simulink model "FT_CAN_messages"  (R2021b)
settings: Solver=FixedStepDiscrete  StartTime=0.0  StopTime=Inf  FixedStep=5e-2  RelTol=1e-3
model workspace (MAT data in the model file):
  MAX_UINT4 = Simulink.Parameter
  MAX_UINT4.Value = 15
  MAX_UINT4.DataType = 'auto'
  MAX_UINT4.Complexity = 'real'
  MAX_UINT4.Dimensions = [1 1]
undefined symbols (not defined in the file): canChannel
libraries: canmsglib x15, canlib x4, slrealtimesharedmemorylib x1, simulink_extras x1
settings Model: Creator=mfussi  LastModifiedBy=ngenesio

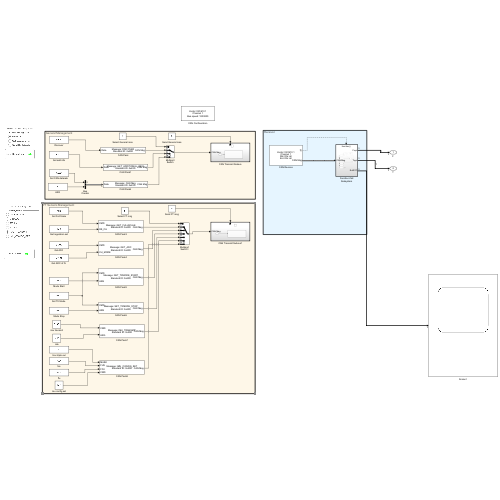
[thumbnail: Simulink's stored preview of the top-level diagram]
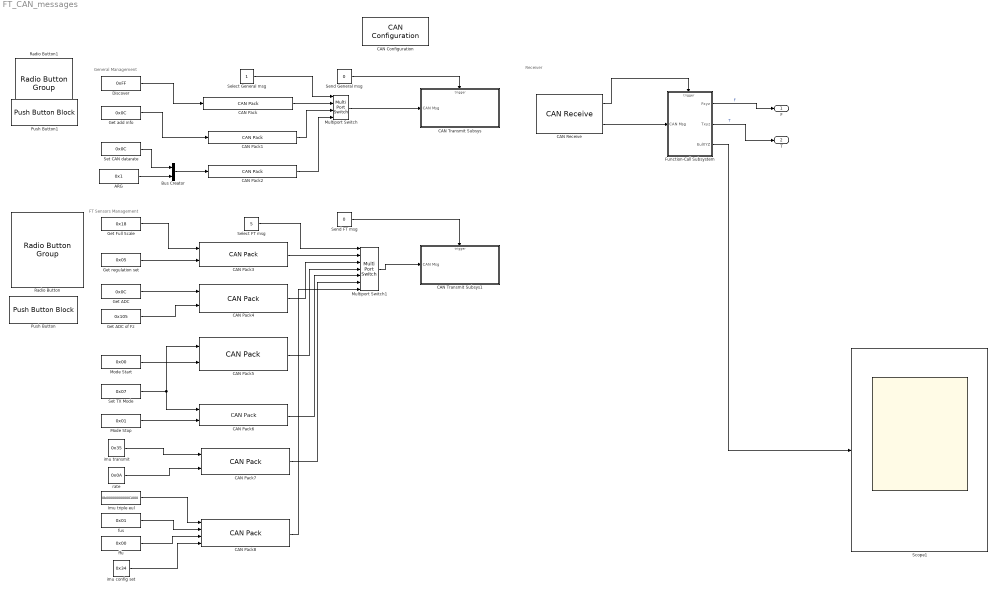
== system FT_CAN_messages ==
  note: Receiver
  note: FT Sensors Management
  note: General Management
  ARG : Constant  Value=0x1  OutDataTypeStr=uint8
  Bus Creator : BusCreator  Inputs=2
  CAN Configuration : canlib/CAN Configuration  BlockHandle=4.0012  Device=Vector VN1610 1 (Channel 1)  DeviceMenu=Vector VN1610 1 (Channel 1)  ObjConstructor=canChannel('Vector', 'VN1610 1', 1)  BusSpeed=1000000  EnableBitParameters=off  SJW=1  TSEG1=4  TSEG2=3  NSamples=1  AckMode=Normal
      settings: SourceProductBaseCode=VN
  CAN Pack : canmsglib/CAN Pack  MsgList=(none)  MsgName=DISCOVER  MsgIDType=Standard (11-bit identifier)  MsgIdentifier=0x20D  MsgLength=1  Remote=off  ApplyMinMax=off  BusOutput=off  SignalInfo={}
      settings: SourceProductBaseCode=ME,XP,VN  DataFormat=raw data
  CAN Pack1 : canmsglib/CAN Pack  MsgList=(none)  MsgName=GET_ADDITIONAL_INFO  MsgIDType=Standard (11-bit identifier)  MsgIdentifier=0x20D  MsgLength=1  Remote=off  ApplyMinMax=off  BusOutput=off  SignalInfo={}
      settings: SourceProductBaseCode=ME,XP,VN  DataFormat=raw data
  CAN Pack2 : canmsglib/CAN Pack  MsgList=(none)  MsgName=CAN Msg  MsgIDType=Standard (11-bit identifier)  MsgIdentifier=0x20D  MsgLength=2  Remote=off  ApplyMinMax=off  BusOutput=off  SignalInfo={}
      settings: SourceProductBaseCode=ME,XP,VN  DataFormat=raw data
  CAN Pack3 : canmsglib/CAN Pack  MsgList=(none)  MsgName=GET_FULLSCALE  MsgIDType=Standard (11-bit identifier)  MsgIdentifier=0x20D  MsgLength=2  Remote=off  ApplyMinMax=off  BusOutput=off  SignalInfo={ 'CMD', '0', '8', 'LE', 'unsigned', 'Standard', '0', '1', '0', '-Inf', 'Inf'; 'RS_CH', '8', '8', 'LE', 'unsigned', 'Standard', '0', '1', '0', '-Inf', 'Inf' }
      settings: SourceProductBaseCode=ME,XP,VN  DataFormat=manually specified signals
  CAN Pack4 : canmsglib/CAN Pack  MsgList=(none)  MsgName=GET_ADC  MsgIDType=Standard (11-bit identifier)  MsgIdentifier=0x20D  MsgLength=3  Remote=off  ApplyMinMax=off  BusOutput=off  SignalInfo={ 'CMD', '0', '8', 'LE', 'unsigned', 'Standard', '0', '1', '0', '-Inf', 'Inf'; 'CH_MODE', '8', '12', 'LE', 'unsigned', 'Standard', '0', '1', '0', '-Inf', 'Inf' }
      settings: SourceProductBaseCode=ME,XP,VN  DataFormat=manually specified signals
  CAN Pack5 : canmsglib/CAN Pack  MsgList=(none)  MsgName=SET_TXMODE_START  MsgIDType=Standard (11-bit identifier)  MsgIdentifier=0x20D  MsgLength=2  Remote=off  ApplyMinMax=off  BusOutput=off  SignalInfo={ 'CMD', '0', '8', 'LE', 'unsigned', 'Standard', '0', '1', '0', '-Inf', 'Inf'; 'ARG', '8', '8', 'LE', 'unsigned', 'Standard', '0', '1', '0', '-Inf', 'Inf' }
      settings: SourceProductBaseCode=ME,XP,VN  DataFormat=manually specified signals
  CAN Pack6 : canmsglib/CAN Pack  MsgList=(none)  MsgName=SET_TXMODE_STOP  MsgIDType=Standard (11-bit identifier)  MsgIdentifier=0x20D  MsgLength=2  Remote=off  ApplyMinMax=off  BusOutput=off  SignalInfo={ 'CMD', '0', '8', 'LE', 'unsigned', 'Standard', '0', '1', '0', '-Inf', 'Inf'; 'ARG', '8', '8', 'LE', 'unsigned', 'Standard', '0', '1', '0', '-Inf', 'Inf' }
      settings: SourceProductBaseCode=ME,XP,VN  DataFormat=manually specified signals
  CAN Pack7 : canmsglib/CAN Pack  MsgList=(none)  MsgName=IMU_TRANSMIT  MsgIDType=Standard (11-bit identifier)  MsgIdentifier=0x20D  MsgLength=8  Remote=off  ApplyMinMax=off  BusOutput=off  SignalInfo={ 'CMD', '0', '8', 'LE', 'unsigned', 'Standard', '0', '1', '0', '-Inf', 'Inf'; 'ARG', '8', '8', 'LE', 'unsigned', 'Standard', '0', '1', '0', '-Inf', 'Inf' }
      settings: SourceProductBaseCode=ME,XP,VN  DataFormat=manually specified signals
  CAN Pack8 : canmsglib/CAN Pack  MsgList=(none)  MsgName=IMU_CONFIG_SET  MsgIDType=Standard (11-bit identifier)  MsgIdentifier=0x20D  MsgLength=8  Remote=off  ApplyMinMax=off  BusOutput=off  SignalInfo={ 'MASK', '8', '16', 'LE', 'unsigned', 'Standard', '0', '1', '0', '-Inf', 'Inf'; 'FUS', '24', '8', 'LE', 'unsigned', 'Standard', '0', '1', '0', '-Inf', 'Inf'; 'FFU', '32', '32', 'LE', 'unsigned', 'Standard', '0', '1', '0', '-Inf', 'Inf'; 'CMD', '0', '8', 'LE', 'unsigned', 'Standard', '0', '1', '0', '-Inf', 'Inf' }
      settings: SourceProductBaseCode=ME,XP,VN  DataFormat=manually specified signals
  CAN Receive : canlib/CAN Receive  BlockHandle=12.0012  Device=Vector VN1610 1 (Channel 1)  DeviceMenu=Vector VN1610 1 (Channel 1)  ObjConstructor=canChannel('Vector', 'VN1610 1', 1)  EnableStandardIDsFilter=off  StdIDsCombo=Allow all  StandardIDs=0  EnableExtendedIDsFilter=off  ExtIDsCombo=Allow all  ExtendedIDs=0  SampleTime=0.1  MsgsPerTimestep=all  InternalFilterUpdateStatus=on  BusOutput=on
      settings: SourceProductBaseCode=VN
  CAN Transmit Subsys : Subsystem  TreatAsAtomicUnit=on
  CAN Transmit Subsys1 : Subsystem  TreatAsAtomicUnit=on
  Discover : Constant  Value=0xFF
  Function-Call Subsystem : Subsystem  TreatAsAtomicUnit=on
  Get ADC : Constant  Value=0x0C  OutDataTypeStr=uint8
  Get ADC of Fz : Constant  Value=0x105  OutDataTypeStr=uint16
  Get Full Scale : Constant  Value=0x18  OutDataTypeStr=uint8
  Get add info : Constant  Value=0x0C
  Get regulation set : Constant  Value=0x05  OutDataTypeStr=uint8
  Imu triple eul : Constant  Value=0b0000000000001000  OutDataTypeStr=uint8
  Mode Start : Constant  Value=0x00  OutDataTypeStr=uint8
  Mode Stop : Constant  Value=0x01  OutDataTypeStr=uint8
  Multiport Switch : MultiPortSwitch
  Multiport Switch1 : MultiPortSwitch  Inputs=6
  Push Button : PushButtonBlock  ButtonText=Send FT Msg  Icon=TurnSignalRight  IconAlignment=Right  IconColor=On  OffValue=0.000000
  Push Button1 : PushButtonBlock  ButtonText=Send General Msg  Icon=TurnSignalRight  IconAlignment=Right  IconColor=On  OffValue=0.000000
  Radio Button : RadioButtonGroup  SelectedLabel=IMU_TRANSMIT  ButtonGroupName=FT Management
      settings: Values={{'Get Full scale', 'Get ADC', 'TX Start', 'TX Stop', 'IMU_TRANSMIT', 'IMU_CONFIG_SET'}, [1 2 3 4 5 6]}
  Radio Button1 : RadioButtonGroup  SelectedLabel=Discover  ButtonGroupName=General Management
      settings: Values={{'Discover', 'Get additional info', 'Set CAN datarate'}, [1 2 3]}
  Scope1 : Scope
  Select FT msg : Constant  Value=5
  Select General msg : Constant
  Send FT msg : Constant  Value=0
  Send General msg : Constant  Value=0
  Set CAN datarate : Constant  Value=0x0C
  "Set TX Mode " : Constant  Value=0x07
  ffu : Constant  Value=0x00  OutDataTypeStr=uint8
  fus : Constant  Value=0x01  OutDataTypeStr=uint8
  imu config set : Constant  Value=0x34
  imu transmit : Constant  Value=0x35
  rate : Constant  Value=0x0A
  F : Outport
  T : Outport  Port=2
  wires:
  Discover/1 -> CAN Pack/1
  CAN Receive/1 -> Function-Call Subsystem/Trigger
  CAN Receive/2 -> Function-Call Subsystem/1(CAN Msg)
  Set CAN datarate/1 -> Bus Creator/1
  ARG/1 -> Bus Creator/2
  Get Full Scale/1 -> CAN Pack3/1
  Get regulation set/1 -> CAN Pack3/2
  Get add info/1 -> CAN Pack1/1
  Bus Creator/1 -> CAN Pack2/1
  Get ADC/1 -> CAN Pack4/1
  Get ADC of Fz/1 -> CAN Pack4/2
  "Set TX Mode "/1 -> CAN Pack5/1, CAN Pack6/1
  Mode Start/1 -> CAN Pack5/2
  Function-Call Subsystem/1(Fxyz) -> F/1  "F"
  Function-Call Subsystem/2(Txyz) -> T/1  "T"
  Select General msg/1 -> Multiport Switch/1
  CAN Pack/1 -> Multiport Switch/2
  CAN Pack1/1 -> Multiport Switch/3
  CAN Pack2/1 -> Multiport Switch/4
  CAN Pack3/1 -> Multiport Switch1/2
  CAN Pack4/1 -> Multiport Switch1/3
  CAN Pack5/1 -> Multiport Switch1/4
  Select FT msg/1 -> Multiport Switch1/1
  Multiport Switch1/1 -> CAN Transmit Subsys1/1(CAN Msg)
  Send FT msg/1 -> CAN Transmit Subsys1/Trigger
  Multiport Switch/1 -> CAN Transmit Subsys/1(CAN Msg)
  Send General msg/1 -> CAN Transmit Subsys/Trigger
  CAN Pack6/1 -> Multiport Switch1/5
  Mode Stop/1 -> CAN Pack6/2
  CAN Pack7/1 -> Multiport Switch1/6
  imu transmit/1 -> CAN Pack7/1
  CAN Pack8/1 -> Multiport Switch1/7
  fus/1 -> CAN Pack8/2
  ffu/1 -> CAN Pack8/3
  Function-Call Subsystem/3(EulXYZ) -> Scope1/1
  rate/1 -> CAN Pack7/2
  imu config set/1 -> CAN Pack8/4
  Imu triple eul/1 -> CAN Pack8/1

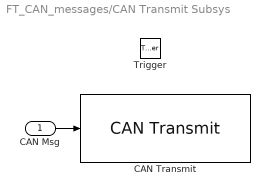
== system FT_CAN_messages/CAN Transmit Subsys ==
  CAN Msg : Inport
  Trigger : TriggerPort  VariantControl=(inherit)
  CAN Transmit : canlib/CAN Transmit  BlockHandle=16.0012  Device=Vector VN1610 1 (Channel 1)  DeviceMenu=Vector VN1610 1 (Channel 1)  ObjConstructor=canChannel('Vector', 'VN1610 1', 1)  EnableEventTransmit=off  EnablePeriodicTransmit=off  MessagePeriod=1.000
      settings: SourceProductBaseCode=VN
  wires:
  CAN Msg/1 -> CAN Transmit/1

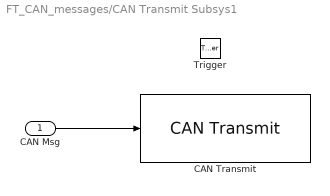
== system FT_CAN_messages/CAN Transmit Subsys1 ==
  CAN Msg : Inport
  Trigger : TriggerPort  VariantControl=(inherit)
  CAN Transmit : canlib/CAN Transmit  BlockHandle=21.0012  Device=Vector VN1610 1 (Channel 1)  DeviceMenu=Vector VN1610 1 (Channel 1)  ObjConstructor=canChannel('Vector', 'VN1610 1', 1)  EnableEventTransmit=off  EnablePeriodicTransmit=off  MessagePeriod=1.000
      settings: SourceProductBaseCode=VN
  wires:
  CAN Msg/1 -> CAN Transmit/1

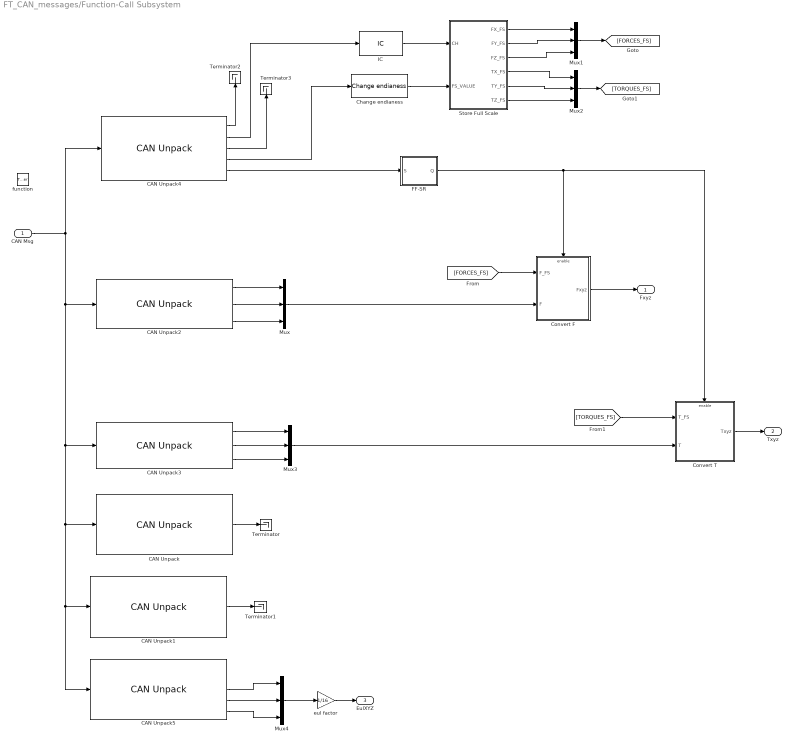
== system FT_CAN_messages/Function-Call Subsystem ==
  CAN Msg : Inport
  function : TriggerPort  TriggerType=function-call  VariantControl=(inherit)
  CAN Unpack : canmsglib/CAN Unpack  MsgList=(none)  MsgName=UNCALIB_F_VECT_DBM  MsgIDType=Standard (11-bit identifier)  MsgIdentifier=0x3D8  MsgLength=6  SignalInfo={}  IDPort=off  TimestampPort=off  ErrorPort=off  RemotePort=off  LengthPort=off  StatusPort=off  ApplyMinMax=off
      settings: SourceProductBaseCode=ME,XP,VN  DataFormat=raw data
  CAN Unpack1 : canmsglib/CAN Unpack  MsgList=(none)  MsgName=UNCALIB_T_VECT_DBM  MsgIDType=Standard (11-bit identifier)  MsgIdentifier=0x3D9  MsgLength=6  SignalInfo={}  IDPort=off  TimestampPort=off  ErrorPort=off  RemotePort=off  LengthPort=off  StatusPort=off  ApplyMinMax=off
      settings: SourceProductBaseCode=ME,XP,VN  DataFormat=raw data
  CAN Unpack2 : canmsglib/CAN Unpack  MsgList=(none)  MsgName=F_VECT  MsgIDType=Standard (11-bit identifier)  MsgIdentifier=0x3DA  MsgLength=6  SignalInfo={ 'FX', '0', '16', 'LE', 'unsigned', 'Standard', '0', '1', '0', '-Inf', 'Inf'; 'FY', '16', '16', 'LE', 'unsigned', 'Standard', '0', '1', '0', '-Inf', 'Inf'; 'FZ', '32', '16', 'LE', 'unsigned', 'Standard', '0', '1', '0', '-Inf', 'Inf' }  IDPort=off  TimestampPort=off  ErrorPort=off  RemotePort=off  LengthPort=off  StatusPort=off  ApplyMinMax=off
      settings: SourceProductBaseCode=ME,XP,VN
  CAN Unpack3 : canmsglib/CAN Unpack  MsgList=(none)  MsgName=T_VECT  MsgIDType=Standard (11-bit identifier)  MsgIdentifier=0x3DB  MsgLength=6  SignalInfo={ 'TX', '0', '16', 'LE', 'unsigned', 'Standard', '0', '1', '0', '-Inf', 'Inf'; 'TY', '16', '16', 'LE', 'unsigned', 'Standard', '0', '1', '0', '-Inf', 'Inf'; 'TZ', '32', '16', 'LE', 'unsigned', 'Standard', '0', '1', '0', '-Inf', 'Inf' }  IDPort=off  TimestampPort=off  ErrorPort=off  RemotePort=off  LengthPort=off  StatusPort=off  ApplyMinMax=off
      settings: SourceProductBaseCode=ME,XP,VN
  CAN Unpack4 : canmsglib/CAN Unpack  MsgList=(none)  MsgName=GET_FULLSCALE  MsgIDType=Standard (11-bit identifier)  MsgIdentifier=0x2D0  MsgLength=4  SignalInfo={ 'CMD', '0', '8', 'LE', 'unsigned', 'Standard', '0', '1', '0', '-Inf', 'Inf'; 'CH', '8', '4', 'LE', 'unsigned', 'Standard', '0', '1', '0', '-Inf', 'Inf'; 'RS', '12', '4', 'LE', 'unsigned', 'Standard', '0', '1', '0', '-Inf', 'Inf'; 'FS', '16', '16', 'LE', 'unsigned', 'Standard', '0', '1', '0', '-Inf', 'Inf' }  IDPort=off  TimestampPort=off  ErrorPort=off  RemotePort=off  LengthPort=off  StatusPort=on  ApplyMinMax=off
      settings: SourceProductBaseCode=ME,XP,VN
  CAN Unpack5 : canmsglib/CAN Unpack  MsgList=(none)  MsgName=IMU_TRIPLE  MsgIDType=Standard (11-bit identifier)  MsgIdentifier=0x5D3  MsgLength=8  SignalInfo={ 'SEQ', '0', '8', 'LE', 'unsigned', 'Standard', '0', '1', '0', '-Inf', 'Inf'; 'SNS', '8', '8', 'LE', 'unsigned', 'Standard', '0', '1', '0', '-Inf', 'Inf'; 'X', '16', '16', 'LE', 'signed', 'Standard', '0', '1', '0', '-Inf', 'Inf'; 'Y', '32', '16', 'LE', 'signed', 'Standard', '0', '1', '0', '-Inf', 'Inf'; 'Z', '48', '16', 'LE', 'signed', 'Standard', '0', '1', '0', '-Inf', 'Inf' }  IDPort=off  TimestampPort=off  ErrorPort=off  RemotePort=off  LengthPort=off  StatusPort=off  ApplyMinMax=off
      settings: SourceProductBaseCode=ME,XP,VN
  Change endianess : slrealtimesharedmemorylib/Change endianess  numInp=1  lengthIn=Byte
      settings: SourceProductBaseCode=XP
  Convert F : Subsystem
  Convert T : Subsystem  TreatAsAtomicUnit=on
  FF-SR : Subsystem
  IC : InitialCondition  Value=MAX_UINT4
  Mux{,1..4} (5 alike) : Mux  Inputs=3
  Store Full Scale : Stateflow chart  TreatAsAtomicUnit=on
  Terminator{,1..3} (4 alike) : Terminator
  eul factor : Gain  Gain=1/16
  Fxyz : Outport  Unit=N  InitialOutput=[0,0,0]
  Txyz : Outport  Port=2  Unit=N*m  InitialOutput=[0,0,0]
  EulXYZ : Outport  Port=3
  wires:
  CAN Msg/1 -> CAN Unpack4/1, CAN Unpack5/1, CAN Unpack1/1, CAN Unpack/1, CAN Unpack3/1, CAN Unpack2/1
  CAN Unpack/1 -> Terminator/1
  CAN Unpack1/1 -> Terminator1/1
  CAN Unpack4/2 -> IC/1
  CAN Unpack4/1 -> Terminator2/1
  IC/1 -> Store Full Scale/1(CH)
  Store Full Scale/1(FX_FS) -> Mux1/1
  Store Full Scale/2(FY_FS) -> Mux1/2
  Store Full Scale/3(FZ_FS) -> Mux1/3
  Convert F/1(Fxyz) -> Fxyz/1
  Store Full Scale/6(TZ_FS) -> Mux2/3
  Store Full Scale/5(TY_FS) -> Mux2/2
  Store Full Scale/4(TX_FS) -> Mux2/1
  Mux1/1 -> [FORCES_FS]
  Mux2/1 -> [TORQUES_FS]
  Convert T/1(Txyz) -> Txyz/1
  CAN Unpack4/3 -> Terminator3/1
  CAN Unpack2/1 -> Mux/1
  CAN Unpack2/2 -> Mux/2
  CAN Unpack2/3 -> Mux/3
  CAN Unpack3/1 -> Mux3/1
  CAN Unpack3/2 -> Mux3/2
  CAN Unpack3/3 -> Mux3/3
  CAN Unpack4/4 -> Change endianess/1
  Mux/1 -> Convert F/2(F)
  Mux3/1 -> Convert T/2(T)
  Change endianess/1 -> Store Full Scale/2(FS_VALUE)
  [TORQUES_FS] -> Convert T/1(T_FS)
  [FORCES_FS] -> Convert F/1(F_FS)
  FF-SR/1(Q) -> Convert F/Enable, Convert T/Enable
  CAN Unpack4/5 -> FF-SR/1(S)
  CAN Unpack5/3 -> Mux4/1
  CAN Unpack5/4 -> Mux4/2
  CAN Unpack5/5 -> Mux4/3
  Mux4/1 -> eul factor/1
  eul factor/1 -> EulXYZ/1

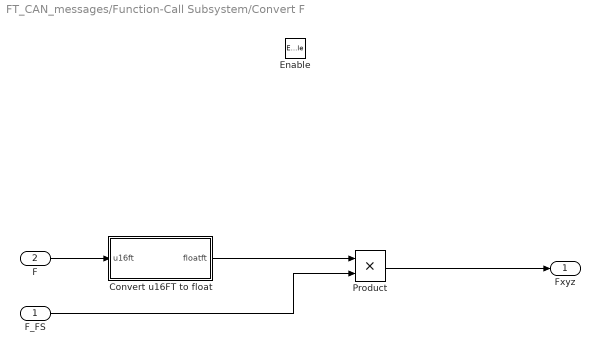
== system FT_CAN_messages/Function-Call Subsystem/Convert F ==
  F_FS : Inport
  F : Inport  Port=2
  Enable : EnablePort
  Convert u16FT to float : Subsystem
  Product : Product  OutDataTypeStr=single
  Fxyz : Outport  OutputWhenDisabled=reset  InitialOutput=[0, 0, 0]
  wires:
  Product/1 -> Fxyz/1
  F_FS/1 -> Product/2
  F/1 -> Convert u16FT to float/1(u16ft)
  Convert u16FT to float/1(floatft) -> Product/1

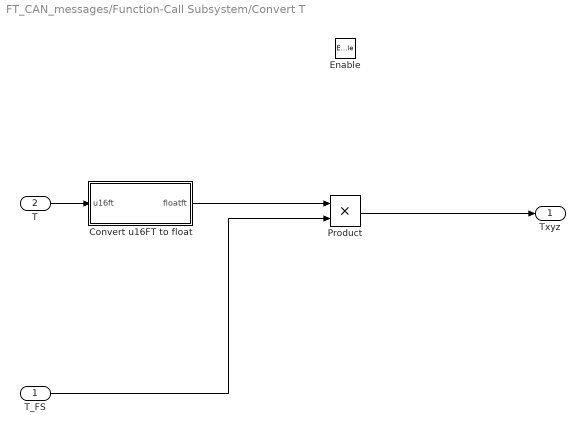
== system FT_CAN_messages/Function-Call Subsystem/Convert T ==
  T_FS : Inport
  T : Inport  Port=2
  Enable : EnablePort
  Convert u16FT to float : Subsystem
  Product : Product
  Txyz : Outport  InitialOutput=[0,0,0]
  wires:
  Product/1 -> Txyz/1
  T/1 -> Convert u16FT to float/1(u16ft)
  T_FS/1 -> Product/2
  Convert u16FT to float/1(floatft) -> Product/1

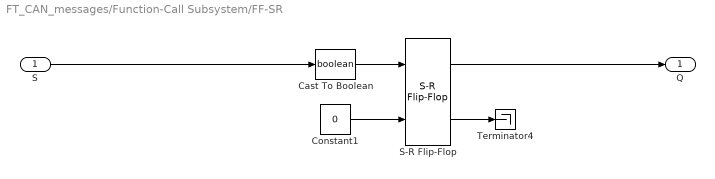
== system FT_CAN_messages/Function-Call Subsystem/FF-SR ==
  S : Inport
  Cast To Boolean : DataTypeConversion  OutDataTypeStr=boolean
  Constant1 : Constant  Value=0  OutDataTypeStr=boolean
  S-R Flip-Flop : simulink_extras/Flip Flops/S-R Flip-Flop  initial_condition=0
  Terminator4 : Terminator
  Q : Outport
  wires:
  S-R Flip-Flop/2 -> Terminator4/1
  Cast To Boolean/1 -> S-R Flip-Flop/1
  Constant1/1 -> S-R Flip-Flop/2
  S-R Flip-Flop/1 -> Q/1
  S/1 -> Cast To Boolean/1

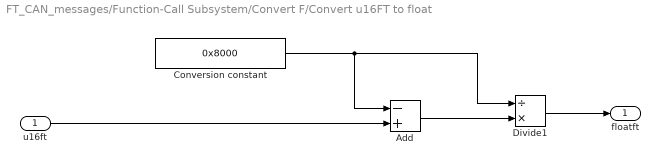
== system FT_CAN_messages/Function-Call Subsystem/Convert F/Convert u16FT to float ==
  u16ft : Inport
  Add : Sum  Inputs=-+  OutDataTypeStr=int16
  Conversion constant : Constant  Value=0x8000  OutDataTypeStr=uint16
  Divide1 : Product  Inputs=/*  OutDataTypeStr=single
  floatft : Outport
  wires:
  u16ft/1 -> Add/2
  Add/1 -> Divide1/2
  Conversion constant/1 -> Add/1, Divide1/1
  Divide1/1 -> floatft/1

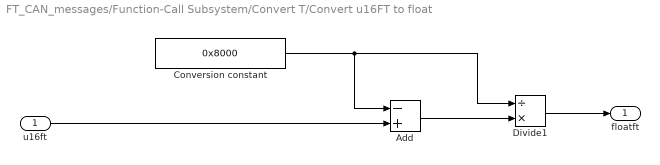
== system FT_CAN_messages/Function-Call Subsystem/Convert T/Convert u16FT to float ==
  u16ft : Inport
  Add : Sum  Inputs=-+  OutDataTypeStr=int16
  Conversion constant : Constant  Value=0x8000  OutDataTypeStr=uint16
  Divide1 : Product  Inputs=/*  OutDataTypeStr=single
  floatft : Outport
  wires:
  u16ft/1 -> Add/2
  Add/1 -> Divide1/2
  Conversion constant/1 -> Add/1, Divide1/1
  Divide1/1 -> floatft/1

== stateflow chart FT_CAN_messages/Function-Call Subsystem/Store Full Scale ==
  note: uint16(0)
  note: uint16(0)
  note: uint16(0)
  state Home
  (junction 45) -> (junction 49) [order 3]
  (junction 49) -> Home [order 1] : [CH==5]
      | {TZ_FS = FS_VALUE;}
  (junction 49) -> Home [order 2] : [CH==4]
      | {TY_FS = FS_VALUE;}
  (default) -> Home
  (junction 45) -> Home [order 1] : [CH==3]
      | {TX_FS = FS_VALUE;}
  (junction 40) -> (junction 45) [order 3]
  (junction 45) -> Home [order 2] : [CH==2]
      | {FZ_FS = FS_VALUE;}
  (junction 40) -> Home [order 1] : [CH==0]
      | {FX_FS = FS_VALUE;}
  Home -> (junction 40) : [CH<=5]
  (junction 40) -> Home [order 2] : [CH==1]
      | {FY_FS = FS_VALUE;}
  data: CH input uint8; FS_VALUE input uint16; FX_FS output uint16 size=1 =uint16(0); FY_FS output uint16 size=1 =uint16(0); FZ_FS output uint16 size=1 =uint16(0); TX_FS output uint16 size=1 =uint16(0); TY_FS output uint16 size=1 =uint16(0); TZ_FS output uint16 size=1 =uint16(0)
